simulink model "Simulink_Model"  (R2025a)
settings: Solver=VariableStepAuto  StartTime=0.0  StopTime=6  RelTol=1e-3
libraries: spsThreePhaseFaultLib x3, spsRMSLib x2, spsGroundLib x1, spsSeriesRLCBranchLib x1, spsThreePhasePISectionLineLib x1, spsThreePhaseParallelRLCLoadLib x1, spsThreePhaseVIMeasurementLib x1, sps_lib x1, spsThreePhaseSourceLib x1
settings Model: Creator=User  LastModifiedBy=User

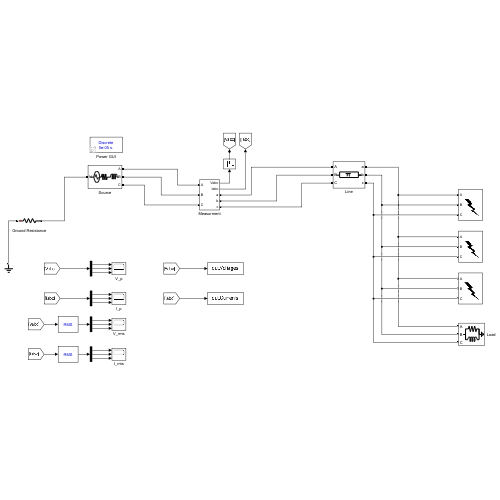
[thumbnail: Simulink's stored preview of the top-level diagram]
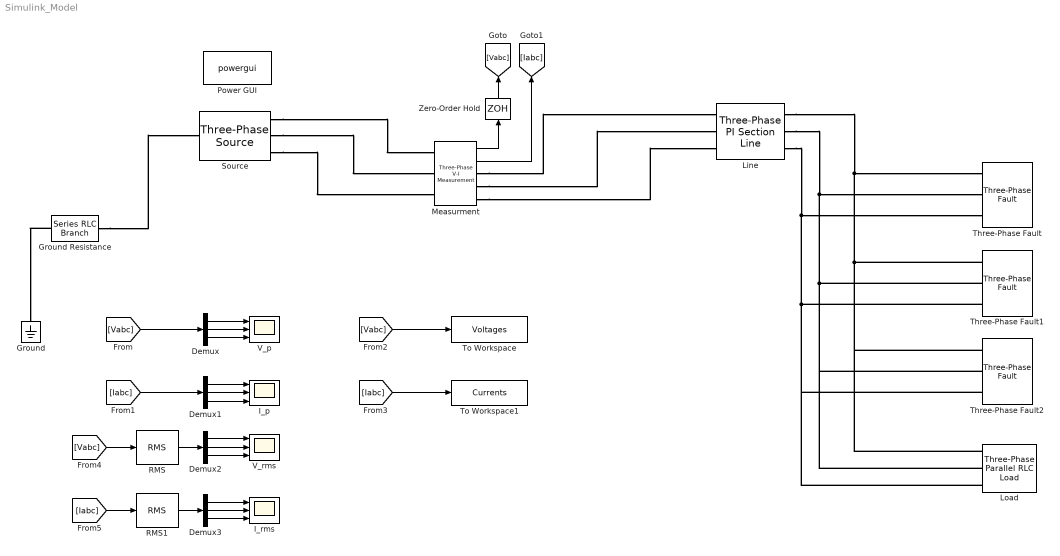
== system Simulink_Model ==
  Demux{,1..3} (4 alike) : Demux  Outputs=3
  Ground : spsGroundLib/Ground  LConnTagsString=a
  Ground Resistance : spsSeriesRLCBranchLib/Series RLC Branch  LConnTagsString=__new0  RConnTagsString=__new0  BranchType=R  Resistance=0.1  Inductance=0  SetiL0=off  InitialCurrent=0  Capacitance=0  Setx0=off  InitialVoltage=0  Measurements=None
  I_p : Scope  NumInputPorts=3
      settings: ActiveDisplayYMinimum=-11210.226374300562  ActiveDisplayYMaximum=11210.226405393661  DataLoggingVariableName=ScopeData2
  I_rms : Scope  NumInputPorts=3
      settings: ActiveDisplayYMinimum=-146.12670109873324  ActiveDisplayYMaximum=2242.2953429330746  DataLoggingVariableName=ScopeData3
  Line : spsThreePhasePISectionLineLib/Three-Phase PI Section Line  LConnTagsString=a|b|c  RConnTagsString=A|B|C  Length=10  Frequency=50  Resistances=[ 0.0115 0.413]  Inductances="[ 1.05e-3  3.32e-3]"  Capacitances=[11.3e-9 5e-9]
  Load : spsThreePhaseParallelRLCLoadLib/Three-Phase Parallel RLC Load  LConnTagsString=A|B|C  Configuration=Y (grounded)  NominalVoltage=11e3  Vabc=[1e3 1e3 1e3]  Vabcp=[1e3 1e3 1e3]  NominalFrequency=50  UnbalancedPower=off  ActivePower=1e6  InductivePower=1e5  CapacitivePower=0  Pabc=[10e3 9e3 11e3]  QLabc=[100 90 110]  QCabc=[100 90 110]  Pabcp=[10e3 9e3 11e3]  QLabcp=[100 90 110]  QCabcp=[100 90 110]  Measurements=None  LoadType=constant Z
  Measurment : spsThreePhaseVIMeasurementLib/Three-Phase V-I Measurement  VoltageMeasurement=phase-to-ground  SetLabelV=off  LabelV=Vabc  Vpu=off  VpuLL=off  CurrentMeasurement=yes  SetLabelI=off  LabelI=Iabc  Ipu=off  Pbase=100e6  Vbase=500e3  OutputType=Complex  PhasorSimulation=off  PSBequivalent=0
  Power GUI : sps_lib/powergui  Priority=1  SimulationMode=Discrete  SampleTime=50e-6  frequency=60  Iterations=50  frequencyindice=50  Pbase=100e6  ErrMax=1e-4  UnitsV=kV  UnitsW=MW  buscounter=0  FunctionMessages=off  echomessages=off  EnableUseOfTLC=off  CurrentSourceSwitches=off  DisableSnubberDevices=off  DisableRonSwitches=off  DisableVfSwitches=off  DisplayEquations=off  AutomaticDiscreteSolvers=off  SolverType=Tustin/Backward Euler (TBE)  Interpol=off  ExternalGateDelay=off  methode=off  Ts=100  x0status=blocks  SPID=on  SwTol=0  HookPort=off  NonlinearTolerance=1e-4  nMaxIteration=100  ContinueOnMaxIteration=off  RestoreLinks=warning  ResistiveCurrentMeasurement=off  Frange=[0:2:500]  Ylog=off  Xlog=on  ShowGrid=off  save=off  variable=ZData  structure=0  ZoomFFT=off  StartTime=0.0  cycles=1  DisplayStyle=1  fundamental=60  FreqAxis=off  MaxFrequency=1000  frequencyindicesteady=1  RmsSteady=1  display=off
  RMS : spsRMSLib/RMS  TrueRMS=on  Freq=50  RMSInit=0  Ts=50e-6
  RMS1 : spsRMSLib/RMS  TrueRMS=on  Freq=60  RMSInit=0  Ts=50e-6
  Source : spsThreePhaseSourceLib/Three-Phase Source  InternalConnection=Yn  VoltagePhases=off  Voltage=11e3  PhaseAngle=0  Voltage_phases=[25e3 25e3 25e3]/sqrt(3)  PhaseAngles_phases=[0 -120 +120]  Frequency=50  NonIdealSource=on  SpecifyImpedance=off  Resistance=0.1  Inductance=0.002  ShortCircuitLevel=100e6  BaseVoltage=11e3  XRratio=7  BusType=swing  Pref=10e3  Qref=0  Prefabc=[10e3, 10e3, 10e3]  Qrefabc=[0, 0, 0]  Qmin=-inf  Qmax=inf
  Three-Phase Fault : spsThreePhaseFaultLib/Three-Phase Fault  InitialStates=0  FaultA=on  FaultB=off  FaultC=off  GroundFault=on  SwitchTimes="[1  1.8]"  External=off  SwitchStatus=NaN  FaultResistance=0.01  GroundResistance=0.001  SnubberResistance=inf  SnubberCapacitance=0  Measurements=None
  Three-Phase Fault1 : spsThreePhaseFaultLib/Three-Phase Fault  InitialStates=0  FaultA=on  FaultB=on  FaultC=off  GroundFault=off  SwitchTimes="[2.5  3.3]"  External=off  SwitchStatus=NaN  FaultResistance=0.01  GroundResistance=0.001  SnubberResistance=inf  SnubberCapacitance=0  Measurements=None
  Three-Phase Fault2 : spsThreePhaseFaultLib/Three-Phase Fault  InitialStates=0  FaultA=on  FaultB=on  FaultC=on  GroundFault=off  SwitchTimes="[4  5]"  External=off  SwitchStatus=NaN  FaultResistance=0.01  GroundResistance=0.001  SnubberResistance=inf  SnubberCapacitance=0  Measurements=None
  To Workspace : ToWorkspace  VariableName=Voltages  SampleTime=-1
  To Workspace1 : ToWorkspace  VariableName=Currents  SampleTime=-1
  V_p : Scope  NumInputPorts=3
      settings: ActiveDisplayYMinimum=-11210.226374300562  ActiveDisplayYMaximum=11210.226405393661
  V_rms : Scope  NumInputPorts=3
      settings: ActiveDisplayYMinimum=-11210.226374300562  ActiveDisplayYMaximum=11210.226405393661
  Zero-Order Hold : ZeroOrderHold  SampleTime=-1
  wires:
  Measurment/1 -> Zero-Order Hold/1
  [Vabc] -> Demux/1
  [Iabc] -> Demux1/1
  Demux/3 -> V_p/3
  Demux1/1 -> I_p/1
  Demux1/2 -> I_p/2
  Demux1/3 -> I_p/3
  [Iabc] -> To Workspace1/1
  [Vabc] -> To Workspace/1
  Zero-Order Hold/1 -> [Vabc]
  Measurment/2 -> [Iabc]
  Demux3/2 -> I_rms/2
  Demux3/1 -> I_rms/1
  Demux2/2 -> V_rms/2
  Demux2/1 -> V_rms/1
  Demux2/3 -> V_rms/3
  [Iabc] -> RMS1/1
  Demux3/3 -> I_rms/3
  [Vabc] -> RMS/1
  RMS/1 -> Demux2/1
  Demux/1 -> V_p/1
  Demux/2 -> V_p/2
  RMS1/1 -> Demux3/1
  connections:
  Ground Resistance/RConn1 -- Source/LConn1
  Ground Resistance/LConn1 -- Ground/LConn1
  Source/RConn1 -- Measurment/LConn1
  Source/RConn2 -- Measurment/LConn2
  Source/RConn3 -- Measurment/LConn3
  Measurment/RConn1 -- Line/LConn1
  Measurment/RConn2 -- Line/LConn2
  Measurment/RConn3 -- Line/LConn3
  Line/RConn1 -- Three-Phase Fault2/LConn1 -- Load/LConn1 -- Three-Phase Fault1/LConn1 -- Three-Phase Fault/LConn1
  Line/RConn2 -- Three-Phase Fault2/LConn2 -- Load/LConn2 -- Three-Phase Fault1/LConn2 -- Three-Phase Fault/LConn2
  Line/RConn3 -- Load/LConn3 -- Three-Phase Fault2/LConn3 -- Three-Phase Fault1/LConn3 -- Three-Phase Fault/LConn3
